simulink model "Practica2_Simulink"  (R2020b)
settings: Solver=VariableStepAuto  StartTime=0.0  StopTime=50  RelTol=1e-3
settings Model: Creator=Danie  LastModifiedBy=Danie

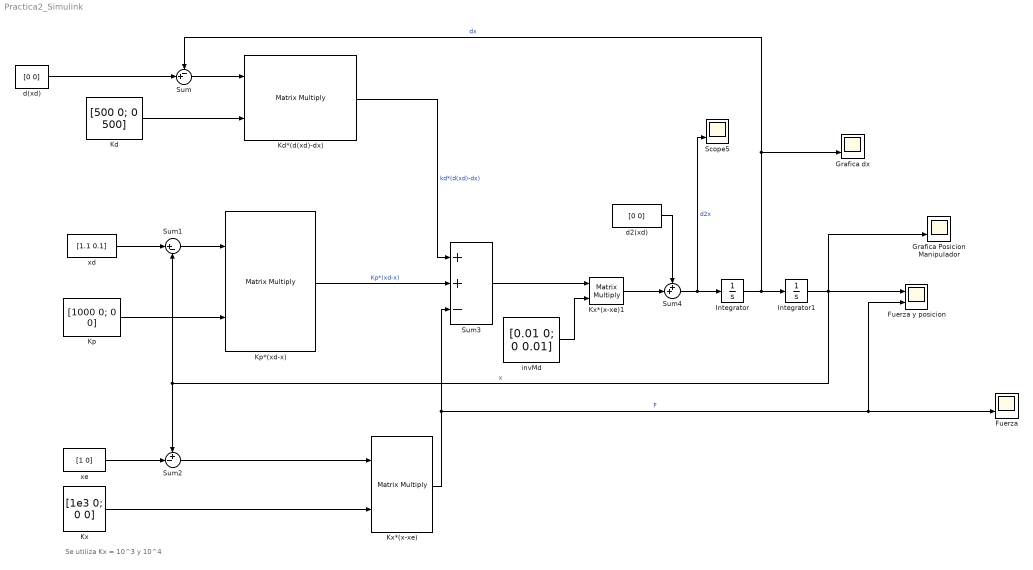
== system Practica2_Simulink ==
  note: Se utiliza Kx = 10^3 y 10^4
  Fuerza : Scope  NumInputPorts=2
  Fuerza y posicion : Scope  NumInputPorts=2
  Grafica Posicion Manipulador : Scope  NumInputPorts=2
  Grafica dx : Scope  NumInputPorts=2
  Integrator : Integrator
  Integrator1 : Integrator
  "Kd " : Constant  Value=[500 0; 0 500]
  "Kd*(d(xd)-dx) " : Product  Multiplication=Matrix(*)
  "Kp " : Constant  Value=[1000 0; 0 0]
  Kp*(xd-x) : Product  Multiplication=Matrix(*)
  Kx : Constant  Value=[1e3 0; 0 0]
  Kx*(x-xe) : Product  Multiplication=Matrix(*)
  "Kx*(x-xe)1 " : Product  Multiplication=Matrix(*)
  Scope5 : Scope  NumInputPorts=2
  Sum : Sum  Inputs=-+|
  Sum1 : Sum  Inputs=|+-
  Sum2 : Sum  Inputs=+-|
  Sum3 : Sum  Inputs=++-
  Sum4 : Sum  Inputs=++|
  "d(xd) " : Constant  Value=[0 0]
  "d2(xd) " : Constant  Value=[0 0]
  "invMd " : Constant  Value=[0.01 0; 0 0.01]
  xd : Constant  Value=[1.1 0.1]
  xe : Constant  Value=[1 0]
  wires:
  Sum3/1 -> "Kx*(x-xe)1 "/1
  Integrator1/1 -> Grafica Posicion Manipulador/2, Sum1/2, Sum2/1, Fuerza y posicion/1  "x"
  Sum2/1 -> Kx*(x-xe)/1
  Sum4/1 -> Scope5/2, Integrator/1  "d2x"
  "d2(xd) "/1 -> Sum4/1
  "Kx*(x-xe)1 "/1 -> Sum4/2
  Kx*(x-xe)/1 -> Sum3/3, Fuerza y posicion/2, Fuerza/2  "F"
  "Kd*(d(xd)-dx) "/1 -> Sum3/1  "kd*(d(xd)-dx)"
  Kx/1 -> Kx*(x-xe)/2
  Sum/1 -> "Kd*(d(xd)-dx) "/1
  Integrator/1 -> Sum/1, Grafica dx/2, Integrator1/1  "dx"
  xe/1 -> Sum2/2
  xd/1 -> Sum1/1
  Kp*(xd-x)/1 -> Sum3/2  "Kp*(xd-x)"
  "Kd "/1 -> "Kd*(d(xd)-dx) "/2
  "invMd "/1 -> "Kx*(x-xe)1 "/2
  Sum1/1 -> Kp*(xd-x)/1
  "Kp "/1 -> Kp*(xd-x)/2
  "d(xd) "/1 -> Sum/2
